simulink model "simpleCarModel"  (R2017a)
settings: Solver=ode45  StartTime=0.0  StopTime=300  MaxStep=0.1  RelTol=1e-3
values from neighbouring files (symbols this model uses):
  A = -1/car_mass*car_rho*car_aero_area*car_cd - car_roll_friction    (= -0.0105939393939)    [initialization.m]
  B = 1/(car_mass*car_tire_rad)    (= 0.0220385674931)    [initialization.m]
  gravity = 9.81    [initialization.m]
  heightmap = [0 1 2 3 4 5 6 7 8 9 10 11 ... (3320 elements, 1660x2)]    [heightmap.mat]    (also in track_heightmap.mat; track_parameters.m = zeros(1660,2))
  Ki = 1/100 * Kp    (= 0.01)    [initialization.m]
  Kp = 1    [initialization.m]
  T_sat = 5    [initialization.m]
  v_d = 25/3.6    (= 6.94444444444)    [initialization.m]
libraries: simulink x1
settings Model: Creator=jorgejac  LastModifiedBy=FF

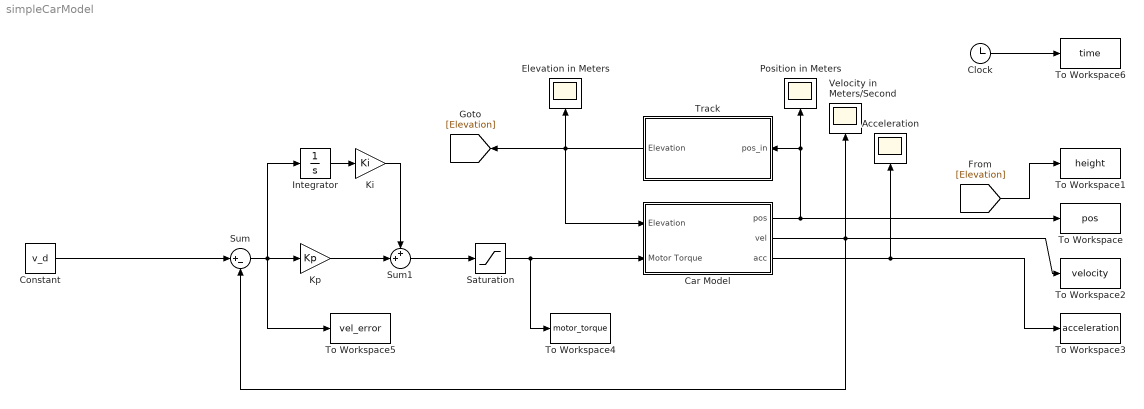
== system simpleCarModel ==
  Acceleration : Scope
  Car Model : Subsystem
  Clock : Clock
  Constant : Constant  Value=v_d
  Elevation in Meters : Scope
  Integrator : Integrator
  Ki : Gain  Gain=Ki
  Kp : Gain  Gain=Kp
  Position in Meters : Scope
  Saturation : Saturate  UpperLimit=T_sat  LowerLimit=-T_sat
  Sum : Sum  Inputs=|+-
  Sum1 : Sum  Inputs=++|
  To Workspace : ToWorkspace  VariableName=pos  SampleTime=-1
  To Workspace1 : ToWorkspace  VariableName=height  SampleTime=-1
  To Workspace2 : ToWorkspace  VariableName=velocity  SampleTime=-1
  To Workspace3 : ToWorkspace  VariableName=acceleration  SampleTime=-1
  To Workspace4 : ToWorkspace  VariableName=motor_torque  SampleTime=-1
  To Workspace5 : ToWorkspace  VariableName=vel_error  SampleTime=-1
  To Workspace6 : ToWorkspace  VariableName=time  SampleTime=-1
  Track : Subsystem
  Velocity in Meters/Second : Scope
  wires:
  Sum1/1 -> Saturation/1
  Car Model/2(vel) -> To Workspace2/1, Sum/2, Velocity in Meters/Second/1
  Car Model/1(pos) -> To Workspace/1, Position in Meters/1, Track/1(pos_in)
  Car Model/3(acc) -> To Workspace3/1, Acceleration/1
  Track/1(Elevation) -> Car Model/1("Elevation "), Elevation in Meters/1, [Elevation]
  [Elevation] -> To Workspace1/1
  Kp/1 -> Sum1/2
  Ki/1 -> Sum1/1
  Integrator/1 -> Ki/1
  Sum/1 -> To Workspace5/1, Integrator/1, Kp/1
  Constant/1 -> Sum/1
  Clock/1 -> To Workspace6/1
  Saturation/1 -> Car Model/2("Motor Torque "), To Workspace4/1

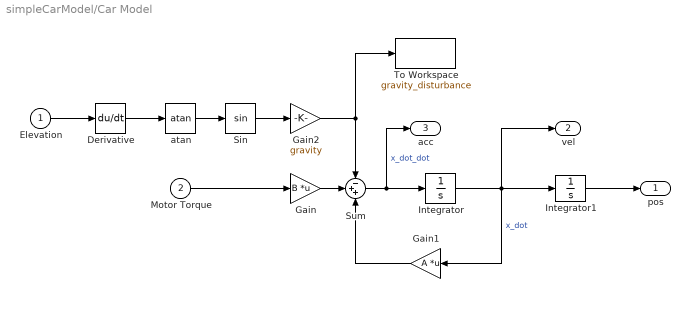
== system simpleCarModel/Car Model ==
  "Elevation " : Inport
  "Motor Torque " : Inport  Port=2
  Derivative : Derivative
  Gain : Gain  Gain=B  Multiplication=Matrix(K*u)
  Gain1 : Gain  Gain=A  Multiplication=Matrix(K*u)
  Gain2 : Gain  Gain=gravity
  Integrator : Integrator
  Integrator1 : Integrator
  Sin : Trigonometry
  Sum : Sum  Inputs=-++
  To Workspace : ToWorkspace  VariableName=gravity_disturbance  SampleTime=-1
  atan : Trigonometry  Operator=atan
  pos : Outport
  vel : Outport  Port=2
  acc : Outport  Port=3
  wires:
  Integrator/1 -> vel/1, Integrator1/1, Gain1/1  "x_dot"
  Gain/1 -> Sum/2
  Sum/1 -> acc/1, Integrator/1  "x_dot_dot"
  Gain1/1 -> Sum/3
  "Motor Torque "/1 -> Gain/1
  Integrator1/1 -> pos/1
  Gain2/1 -> To Workspace/1, Sum/1
  "Elevation "/1 -> Derivative/1
  Derivative/1 -> atan/1
  atan/1 -> Sin/1
  Sin/1 -> Gain2/1

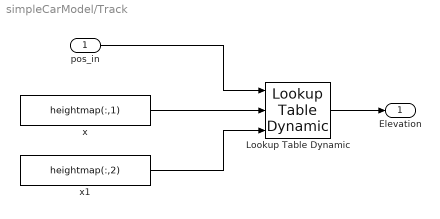
== system simpleCarModel/Track ==
  pos_in : Inport
  Lookup Table Dynamic : simulink/Lookup Tables/Lookup Table Dynamic  LookUpMeth=Interpolation-Use End Values  OutDataType=fixdt('double')  OutScaling=[]  OutputDataTypeScalingMode=Specify via dialog  OutDataTypeStr=double  DoSatur=off
      settings: SourceProductName=Simulink
  x : Constant  Value=heightmap(:,1)
  x1 : Constant  Value=heightmap(:,2)  VectorParams1D=off
  Elevation : Outport
  wires:
  pos_in/1 -> Lookup Table Dynamic/1
  Lookup Table Dynamic/1 -> Elevation/1
  x1/1 -> Lookup Table Dynamic/3
  x/1 -> Lookup Table Dynamic/2
